simulink model "controller"  (R2024b)
settings: Solver=ode4  StartTime=0.0  StopTime=4  FixedStep=0.001  RelTol=1e-3
undefined symbols (not defined in the file): param
libraries: slpidlib x4
settings Model: Creator=mirkomizzoni  LastModifiedBy=mirkomizzoni

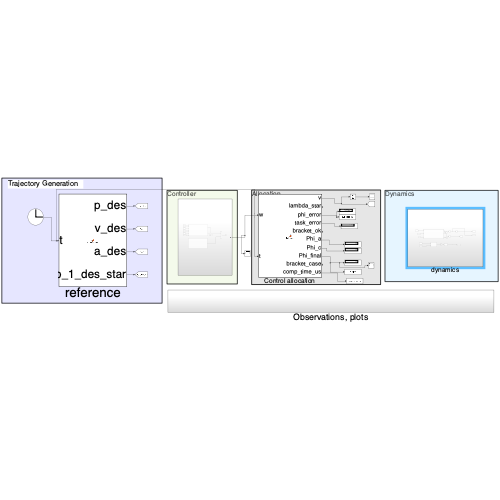
[thumbnail: Simulink's stored preview of the top-level diagram]
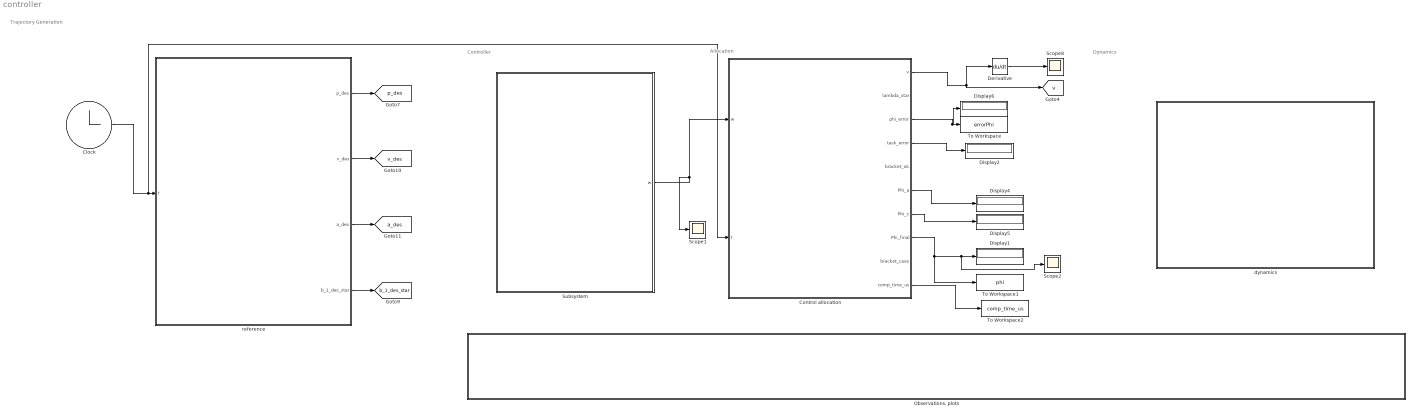
== system controller ==
  note: Trajectory Generation
  note: Dynamics
  note: Allocation
  note: Controller
  Clock : Clock
  Control allocation : MATLAB Function  TreatAsAtomicUnit=on
  Derivative : Derivative
  Display{1..2,4..6} (5 alike) : Display
  "Observations, plots" : Subsystem
  Scope1 : Scope
  Scope2 : Scope
  Scope8 : Scope
  Subsystem : Subsystem
  To Workspace : ToWorkspace  VariableName=errorPhi  SampleTime=-1
  To Workspace1 : ToWorkspace  VariableName=phi  SampleTime=-1
  To Workspace2 : ToWorkspace  VariableName=comp_time_us  SampleTime=-1
      settings: Save2DSignal=2-D array (concatenate along first dimension)
  dynamics : Subsystem
  reference : MATLAB Function  TreatAsAtomicUnit=on
  tag scope: a_des=global, b_1_des_star=global, p_des=global, v=global, v_des=global
  wires:
  reference/1(p_des) -> [p_des]
  Clock/1 -> Control allocation/2(t), reference/1(t)
  reference/3(a_des) -> [a_des]
  reference/4(b_1_des_star) -> [b_1_des_star]
  reference/2(v_des) -> [v_des]
  Control allocation/1(v) -> Derivative/1, [v]
  Derivative/1 -> Scope8/1
  Subsystem/1(w) -> Scope1/1, Control allocation/1(w)
  Control allocation/3(phi_error) -> Display6/1, To Workspace/1
  Control allocation/6(Phi_a) -> Display4/1
  Control allocation/7(Phi_c) -> Display5/1
  Control allocation/4(task_error) -> Display2/1
  Control allocation/8(Phi_final) -> To Workspace1/1, Scope2/1, Display1/1
  Control allocation/10(comp_time_us) -> To Workspace2/1

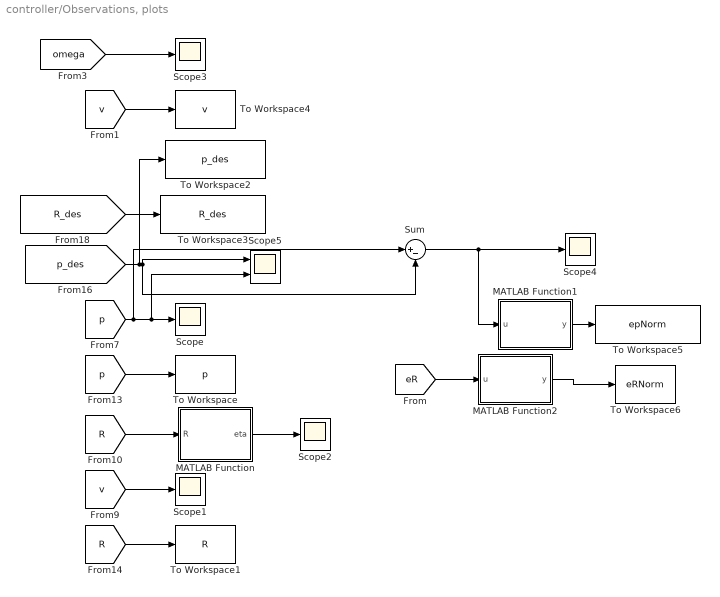
== system controller/Observations, plots ==
  MATLAB Function : MATLAB Function  TreatAsAtomicUnit=on
  MATLAB Function1 : MATLAB Function  TreatAsAtomicUnit=on
  MATLAB Function2 : MATLAB Function  TreatAsAtomicUnit=on
  Scope{,1..4} (5 alike) : Scope
  Scope5 : Scope  NumInputPorts=2
  Sum : Sum  Inputs=|+-
  To Workspace : ToWorkspace  VariableName=p  SampleTime=-1
  To Workspace1 : ToWorkspace  VariableName=R  SaveFormat=Timeseries  SampleTime=-1
  To Workspace2 : ToWorkspace  VariableName=p_des  SampleTime=-1
  To Workspace3 : ToWorkspace  VariableName=R_des  SaveFormat=Timeseries  SampleTime=-1
  To Workspace4 : ToWorkspace  VariableName=v  SampleTime=-1
  To Workspace5 : ToWorkspace  VariableName=epNorm  SampleTime=-1
  To Workspace6 : ToWorkspace  VariableName=eRNorm  SaveFormat=Timeseries  SampleTime=-1
  wires:
  [v] -> Scope1/1
  [R] -> MATLAB Function/1(R)
  [p] -> To Workspace/1
  MATLAB Function/1(eta) -> Scope2/1
  [p] -> Sum/1, Scope/1, Scope5/2
  [R] -> To Workspace1/1
  [p_des] -> Scope5/1, Sum/2, To Workspace2/1
  [R_des] -> To Workspace3/1
  [v] -> To Workspace4/1
  [omega] -> Scope3/1
  Sum/1 -> MATLAB Function1/1(u), Scope4/1
  MATLAB Function1/1(y) -> To Workspace5/1
  MATLAB Function2/1(y) -> To Workspace6/1
  [eR] -> MATLAB Function2/1(u)

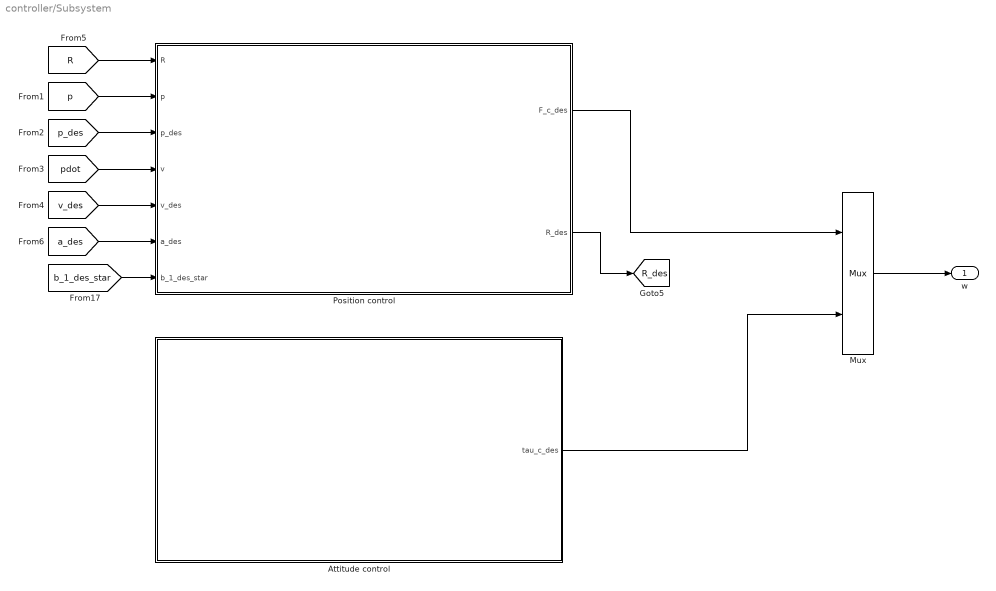
== system controller/Subsystem ==
  Attitude control : Subsystem
  Mux : Mux  Inputs=2
  Position control : Subsystem
  w : Outport
  tag scope: R_des=global
  wires:
  Position control/1(F_c_des) -> Mux/1
  Attitude control/1(tau_c_des) -> Mux/2
  [p_des] -> Position control/3(p_des)
  Position control/2(R_des) -> [R_des]
  [b_1_des_star] -> Position control/7(b_1_des_star)
  [p] -> Position control/2(p)
  [pdot] -> Position control/4(v)
  [R] -> Position control/1(R)
  Mux/1 -> w/1
  [v_des] -> Position control/5(v_des)
  [a_des] -> Position control/6(a_des)

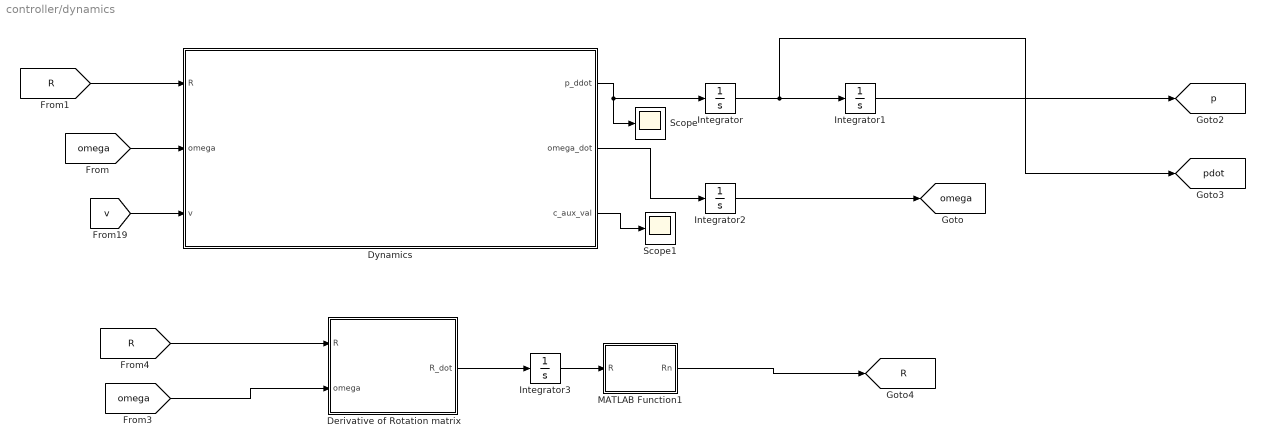
== system controller/dynamics ==
  Derivative of Rotation matrix : MATLAB Function  TreatAsAtomicUnit=on
  Dynamics : MATLAB Function  TreatAsAtomicUnit=on
  Integrator : Integrator  InitialCondition=zeros(3, 1)
  Integrator1 : Integrator  InitialCondition=[0;0.5;0]
  Integrator2 : Integrator  InitialCondition=zeros(3, 1)
  Integrator3 : Integrator  InitialCondition=param.R0
  MATLAB Function1 : MATLAB Function  TreatAsAtomicUnit=on
  Scope : Scope
  Scope1 : Scope
  tag scope: R=global, omega=global, p=global, pdot=global
  wires:
  Derivative of Rotation matrix/1(R_dot) -> Integrator3/1
  [omega] -> Dynamics/2(omega)
  Integrator2/1 -> [omega]
  Dynamics/1(p_ddot) -> Scope/1, Integrator/1
  Integrator1/1 -> [p]
  Integrator/1 -> [pdot], Integrator1/1
  Dynamics/2(omega_dot) -> Integrator2/1
  [R] -> Derivative of Rotation matrix/1(R)
  [R] -> Dynamics/1(R)
  Dynamics/3(c_aux_val) -> Scope1/1
  [v] -> Dynamics/3(v)
  Integrator3/1 -> MATLAB Function1/1(R)
  [omega] -> Derivative of Rotation matrix/2(omega)
  MATLAB Function1/1(Rn) -> [R]

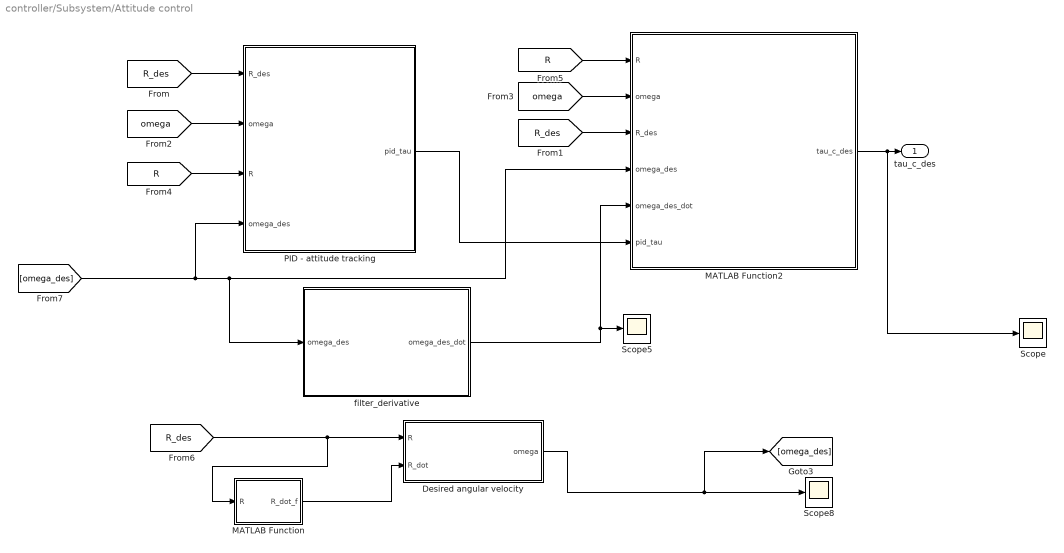
== system controller/Subsystem/Attitude control ==
  Desired angular velocity : MATLAB Function  TreatAsAtomicUnit=on
  MATLAB Function : MATLAB Function  TreatAsAtomicUnit=on
  MATLAB Function2 : MATLAB Function  TreatAsAtomicUnit=on
  PID - attitude tracking : Subsystem
  Scope : Scope
  Scope5 : Scope
  Scope8 : Scope
  filter_derivative : MATLAB Function  TreatAsAtomicUnit=on
  tau_c_des : Outport
  wires:
  MATLAB Function/1(R_dot_f) -> Desired angular velocity/2(R_dot)
  PID - attitude tracking/1(pid_tau) -> MATLAB Function2/6(pid_tau)
  MATLAB Function2/1(tau_c_des) -> Scope/1, tau_c_des/1
  filter_derivative/1(omega_des_dot) -> MATLAB Function2/5(omega_des_dot), Scope5/1
  [R_des] -> PID - attitude tracking/1(R_des)
  [R_des] -> MATLAB Function2/3(R_des)
  [omega] -> PID - attitude tracking/2(omega)
  [omega] -> MATLAB Function2/2(omega)
  [R] -> PID - attitude tracking/3(R)
  [R] -> MATLAB Function2/1(R)
  [R_des] -> MATLAB Function/1(R), Desired angular velocity/1(R)
  Desired angular velocity/1(omega) -> Scope8/1, [omega_des]
  [omega_des] -> PID - attitude tracking/4(omega_des), filter_derivative/1(omega_des), MATLAB Function2/4(omega_des)

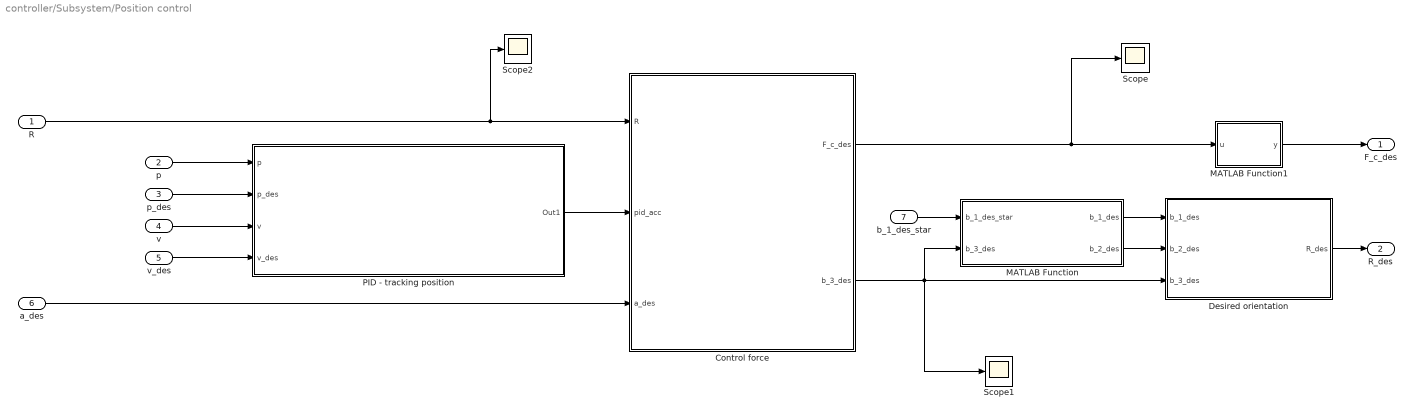
== system controller/Subsystem/Position control ==
  R : Inport
  p : Inport  Port=2
  p_des : Inport  Port=3
  v : Inport  Port=4
  v_des : Inport  Port=5
  a_des : Inport  Port=6
  b_1_des_star : Inport  Port=7
  Control force : MATLAB Function  TreatAsAtomicUnit=on
  Desired orientation : MATLAB Function  TreatAsAtomicUnit=on
  MATLAB Function : MATLAB Function  TreatAsAtomicUnit=on
  MATLAB Function1 : MATLAB Function  TreatAsAtomicUnit=on
  PID - tracking position : Subsystem
  Scope : Scope
  Scope1 : Scope
  Scope2 : Scope
  F_c_des : Outport
  R_des : Outport  Port=2
  wires:
  Control force/1(F_c_des) -> Scope/1, MATLAB Function1/1(u)
  Control force/2(b_3_des) -> Scope1/1, Desired orientation/3(b_3_des), MATLAB Function/2(b_3_des)
  R/1 -> Scope2/1, Control force/1(R)
  p_des/1 -> PID - tracking position/2(p_des)
  Desired orientation/1(R_des) -> R_des/1
  p/1 -> PID - tracking position/1(p)
  v_des/1 -> PID - tracking position/4(v_des)
  a_des/1 -> Control force/3(a_des)
  v/1 -> PID - tracking position/3(v)
  PID - tracking position/1(Out1) -> Control force/2(pid_acc)
  MATLAB Function/1(b_1_des) -> Desired orientation/1(b_1_des)
  MATLAB Function/2(b_2_des) -> Desired orientation/2(b_2_des)
  b_1_des_star/1 -> MATLAB Function/1(b_1_des_star)
  MATLAB Function1/1(y) -> F_c_des/1

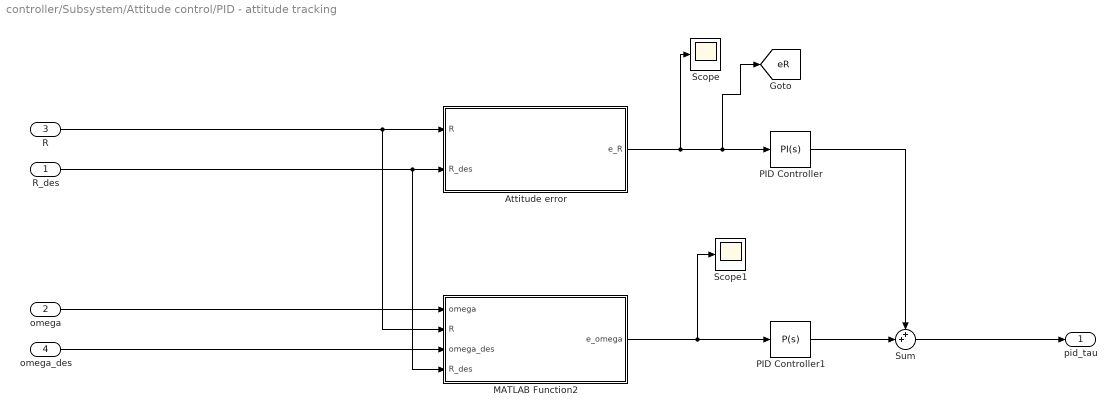
== system controller/Subsystem/Attitude control/PID - attitude tracking ==
  R_des : Inport
  omega : Inport  Port=2
  R : Inport  Port=3
  omega_des : Inport  Port=4
  Attitude error : MATLAB Function  TreatAsAtomicUnit=on
  MATLAB Function2 : MATLAB Function  TreatAsAtomicUnit=on
  PID Controller : slpidlib/PID Controller  Controller=PI  Form=Parallel  TimeDomain=Continuous-time  UseExternalTs=off  SampleTime=-1  IntegratorMethod=Forward Euler  FilterMethod=Forward Euler  ControllerParametersSource=internal  P=4*diag(param.K_tau_p)  I=[0;0;0]  UseKiTs=off  D=0  UseExternalDerivativeSource=off  N=100  UseFilter=on  TunerSelectOption=Transfer Function Based (PID Tuner App)  InitialConditionSource=internal  InitialConditionForIntegrator=0  InitialConditionForFilter=0  DifferentiatorICPrevScaledInput=0  ExternalReset=none  TrackingMode=off  Kt=1  LimitOutput=off  SatLimitsSource=internal  UpperSaturationLimit=inf  LowerSaturationLimit=-inf  LinearizeAsGain=on  AntiWindupMode=none  Kb=1  LimitIntegrator=off  UpperIntegratorSaturationLimit=inf  LowerIntegratorSaturationLimit=-inf  POutMin=[]  POutMax=[]  IOutMin=[]  IOutMax=[]  DOutMin=[]  DOutMax=[]  NOutMin=[]  NOutMax=[]  SumOutMin=[]  SumOutMax=[]  SaturationOutMin=[]  SaturationOutMax=[]  PParamMin=[]  PParamMax=[]  IParamMin=[]  IParamMax=[]  DParamMin=[]  DParamMax=[]  NParamMin=[]  NParamMax=[]  KbParamMin=[]  KbParamMax=[]  KtParamMin=[]  KtParamMax=[]  KbOutMin=[]  KbOutMax=[]  KtOutMin=[]  KtOutMax=[]  IntegratorOutMin=[]  IntegratorOutMax=[]  FilterOutMin=[]  FilterOutMax=[]  SumI1OutMin=[]  SumI1OutMax=[]  SumI2OutMin=[]  SumI2OutMax=[]  SumI3OutMin=[]  SumI3OutMax=[]  SumI4OutMin=[]  SumI4OutMax=[]  SumDOutMin=[]  SumDOutMax=[]  DifferentiatorOutMin=[]  DifferentiatorOutMax=[]  FilterDiffOutCoefMin=[]  FilterDiffOutCoefMax=[]  ReciprocalOutMin=[]  ReciprocalOutMax=[]  SumDenOutMin=[]  SumDenOutMax=[]  SumNumOutMin=[]  SumNumOutMax=[]  DivideOutMin=[]  DivideOutMax=[]  UdiffTsProdOutMin=[]  UdiffTsProdOutMax=[]  NTsProdOutMin=[]  NTsProdOutMax=[]  UintegralTsProdOutMin=[]  UintegralTsProdOutMax=[]  UngainTsProdOutMin=[]  UngainTsProdOutMax=[]  ClampingZeroOutDataTypeStr=Inherit: Inherit via back propagation  ClampingZeroOutMin=[]  ClampingZeroOutMax=[]  FilterDenConstantOutDataTypeStr=Inherit: Inherit via back propagation  FilterDenConstantOutMin=[]  FilterDenConstantOutMax=[]  PCopyOutDataTypeStr=Inherit: Inherit via back propagation  PCopyOutMin=[]  PCopyOutMax=[]  NCopyOutDataTypeStr=Inherit: Inherit via back propagation  NCopyOutMin=[]  NCopyOutMax=[]  IntegratorContinuousStateAttributes=''  IntegratorStateMustResolveToSignalObject=off  IntegratorRTWStateStorageClass=Auto  FilterContinuousStateAttributes=''  FilterStateMustResolveToSignalObject=off  FilterRTWStateStorageClass=Auto  ParallelPVariant=InternalParameters  IdealPVariant=Disabled  IVariant=InternalParameters  DVariant=Disabled  IntegratorVariant=Continuous  SatVariant=Disabled  AWVariant=Passthrough  PCopyVariant=Disabled  TRVariant=Disabled  FdbkBlocksVariant=Forward  IdealPFdbkVariant=Disabled  SatFdbkVariant=Disabled  DerivativeFilterVariant=Disabled  NVariant=Disabled  NCopyVariant=Disabled_SignalSpec  FilterICVariant=Disabled  IntegratorICVariant=InternalICs  ExternalResetVariant=Disabled  TRSumVariant=Passthrough  SumFdbkVariant=Disabled  SumVariant=Sum_PI  TsampFilterVariant=InternalTs  TsampNgainVariant=Passthrough  TsampIntegralVariant=Disabled_SignalSpec  ExternalSaturationOutDataTypeStr=Inherit: Same as second input  DerivativeSourceVariant=Disabled  PreIntVariant=InternalPreInt
  PID Controller1 : slpidlib/PID Controller  Controller=P  Form=Parallel  TimeDomain=Continuous-time  UseExternalTs=off  SampleTime=-1  IntegratorMethod=Forward Euler  FilterMethod=Forward Euler  ControllerParametersSource=internal  P=10*diag(param.K_tau_d)  I=1  UseKiTs=off  D=0  UseExternalDerivativeSource=off  N=100  UseFilter=on  TunerSelectOption=Transfer Function Based (PID Tuner App)  InitialConditionSource=internal  InitialConditionForIntegrator=0  InitialConditionForFilter=0  DifferentiatorICPrevScaledInput=0  ExternalReset=none  TrackingMode=off  Kt=1  LimitOutput=off  SatLimitsSource=internal  UpperSaturationLimit=inf  LowerSaturationLimit=-inf  LinearizeAsGain=on  AntiWindupMode=none  Kb=1  LimitIntegrator=off  UpperIntegratorSaturationLimit=inf  LowerIntegratorSaturationLimit=-inf  POutMin=[]  POutMax=[]  IOutMin=[]  IOutMax=[]  DOutMin=[]  DOutMax=[]  NOutMin=[]  NOutMax=[]  SumOutMin=[]  SumOutMax=[]  SaturationOutMin=[]  SaturationOutMax=[]  PParamMin=[]  PParamMax=[]  IParamMin=[]  IParamMax=[]  DParamMin=[]  DParamMax=[]  NParamMin=[]  NParamMax=[]  KbParamMin=[]  KbParamMax=[]  KtParamMin=[]  KtParamMax=[]  KbOutMin=[]  KbOutMax=[]  KtOutMin=[]  KtOutMax=[]  IntegratorOutMin=[]  IntegratorOutMax=[]  FilterOutMin=[]  FilterOutMax=[]  SumI1OutMin=[]  SumI1OutMax=[]  SumI2OutMin=[]  SumI2OutMax=[]  SumI3OutMin=[]  SumI3OutMax=[]  SumI4OutMin=[]  SumI4OutMax=[]  SumDOutMin=[]  SumDOutMax=[]  DifferentiatorOutMin=[]  DifferentiatorOutMax=[]  FilterDiffOutCoefMin=[]  FilterDiffOutCoefMax=[]  ReciprocalOutMin=[]  ReciprocalOutMax=[]  SumDenOutMin=[]  SumDenOutMax=[]  SumNumOutMin=[]  SumNumOutMax=[]  DivideOutMin=[]  DivideOutMax=[]  UdiffTsProdOutMin=[]  UdiffTsProdOutMax=[]  NTsProdOutMin=[]  NTsProdOutMax=[]  UintegralTsProdOutMin=[]  UintegralTsProdOutMax=[]  UngainTsProdOutMin=[]  UngainTsProdOutMax=[]  ClampingZeroOutDataTypeStr=Inherit: Inherit via back propagation  ClampingZeroOutMin=[]  ClampingZeroOutMax=[]  FilterDenConstantOutDataTypeStr=Inherit: Inherit via back propagation  FilterDenConstantOutMin=[]  FilterDenConstantOutMax=[]  PCopyOutDataTypeStr=Inherit: Inherit via back propagation  PCopyOutMin=[]  PCopyOutMax=[]  NCopyOutDataTypeStr=Inherit: Inherit via back propagation  NCopyOutMin=[]  NCopyOutMax=[]  IntegratorContinuousStateAttributes=''  IntegratorStateMustResolveToSignalObject=off  IntegratorRTWStateStorageClass=Auto  FilterContinuousStateAttributes=''  FilterStateMustResolveToSignalObject=off  FilterRTWStateStorageClass=Auto  ParallelPVariant=InternalParameters  IdealPVariant=Disabled  IVariant=Disabled  DVariant=Disabled  IntegratorVariant=Disabled  SatVariant=Disabled  AWVariant=Disabled  PCopyVariant=Disabled  TRVariant=Disabled  FdbkBlocksVariant=Forward  IdealPFdbkVariant=Disabled  SatFdbkVariant=Disabled  DerivativeFilterVariant=Disabled  NVariant=Disabled  NCopyVariant=Disabled_SignalSpec  FilterICVariant=Disabled  IntegratorICVariant=Disabled  ExternalResetVariant=Disabled  TRSumVariant=Passthrough  SumFdbkVariant=Disabled  SumVariant=Passthrough_P  TsampFilterVariant=InternalTs  TsampNgainVariant=Passthrough  TsampIntegralVariant=Disabled_SignalSpec  ExternalSaturationOutDataTypeStr=Inherit: Same as second input  DerivativeSourceVariant=Disabled  PreIntVariant=InternalPreInt
  Scope : Scope
  Scope1 : Scope
  Sum : Sum  Inputs=++|
  pid_tau : Outport
  tag scope: eR=global
  wires:
  omega/1 -> MATLAB Function2/1(omega)
  omega_des/1 -> MATLAB Function2/3(omega_des)
  PID Controller1/1 -> Sum/2
  Sum/1 -> pid_tau/1
  Attitude error/1(e_R) -> Scope/1, [eR], PID Controller/1
  MATLAB Function2/1(e_omega) -> Scope1/1, PID Controller1/1
  R/1 -> Attitude error/1(R), MATLAB Function2/2(R)
  PID Controller/1 -> Sum/1
  R_des/1 -> Attitude error/2(R_des), MATLAB Function2/4(R_des)

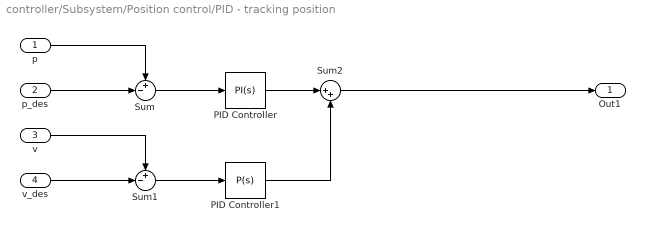
== system controller/Subsystem/Position control/PID - tracking position ==
  p : Inport
  p_des : Inport  Port=2
  v : Inport  Port=3
  v_des : Inport  Port=4
  PID Controller : slpidlib/PID Controller  Controller=PI  Form=Parallel  TimeDomain=Continuous-time  UseExternalTs=off  SampleTime=-1  IntegratorMethod=Forward Euler  FilterMethod=Forward Euler  ControllerParametersSource=internal  P=diag(param.K_F_p)  I=0*diag(param.K_F_i)  UseKiTs=off  D=0  UseExternalDerivativeSource=off  N=100  UseFilter=on  TunerSelectOption=Transfer Function Based (PID Tuner App)  InitialConditionSource=internal  InitialConditionForIntegrator=0  InitialConditionForFilter=0  DifferentiatorICPrevScaledInput=0  ExternalReset=none  TrackingMode=off  Kt=1  LimitOutput=off  SatLimitsSource=internal  UpperSaturationLimit=inf  LowerSaturationLimit=-inf  LinearizeAsGain=on  AntiWindupMode=none  Kb=1  LimitIntegrator=off  UpperIntegratorSaturationLimit=inf  LowerIntegratorSaturationLimit=-inf  POutMin=[]  POutMax=[]  IOutMin=[]  IOutMax=[]  DOutMin=[]  DOutMax=[]  NOutMin=[]  NOutMax=[]  SumOutMin=[]  SumOutMax=[]  SaturationOutMin=[]  SaturationOutMax=[]  PParamMin=[]  PParamMax=[]  IParamMin=[]  IParamMax=[]  DParamMin=[]  DParamMax=[]  NParamMin=[]  NParamMax=[]  KbParamMin=[]  KbParamMax=[]  KtParamMin=[]  KtParamMax=[]  KbOutMin=[]  KbOutMax=[]  KtOutMin=[]  KtOutMax=[]  IntegratorOutMin=[]  IntegratorOutMax=[]  FilterOutMin=[]  FilterOutMax=[]  SumI1OutMin=[]  SumI1OutMax=[]  SumI2OutMin=[]  SumI2OutMax=[]  SumI3OutMin=[]  SumI3OutMax=[]  SumI4OutMin=[]  SumI4OutMax=[]  SumDOutMin=[]  SumDOutMax=[]  DifferentiatorOutMin=[]  DifferentiatorOutMax=[]  FilterDiffOutCoefMin=[]  FilterDiffOutCoefMax=[]  ReciprocalOutMin=[]  ReciprocalOutMax=[]  SumDenOutMin=[]  SumDenOutMax=[]  SumNumOutMin=[]  SumNumOutMax=[]  DivideOutMin=[]  DivideOutMax=[]  UdiffTsProdOutMin=[]  UdiffTsProdOutMax=[]  NTsProdOutMin=[]  NTsProdOutMax=[]  UintegralTsProdOutMin=[]  UintegralTsProdOutMax=[]  UngainTsProdOutMin=[]  UngainTsProdOutMax=[]  ClampingZeroOutDataTypeStr=Inherit: Inherit via back propagation  ClampingZeroOutMin=[]  ClampingZeroOutMax=[]  FilterDenConstantOutDataTypeStr=Inherit: Inherit via back propagation  FilterDenConstantOutMin=[]  FilterDenConstantOutMax=[]  PCopyOutDataTypeStr=Inherit: Inherit via back propagation  PCopyOutMin=[]  PCopyOutMax=[]  NCopyOutDataTypeStr=Inherit: Inherit via back propagation  NCopyOutMin=[]  NCopyOutMax=[]  IntegratorContinuousStateAttributes=''  IntegratorStateMustResolveToSignalObject=off  IntegratorRTWStateStorageClass=Auto  FilterContinuousStateAttributes=''  FilterStateMustResolveToSignalObject=off  FilterRTWStateStorageClass=Auto  ParallelPVariant=InternalParameters  IdealPVariant=Disabled  IVariant=InternalParameters  DVariant=Disabled  IntegratorVariant=Continuous  SatVariant=Disabled  AWVariant=Passthrough  PCopyVariant=Disabled  TRVariant=Disabled  FdbkBlocksVariant=Forward  IdealPFdbkVariant=Disabled  SatFdbkVariant=Disabled  DerivativeFilterVariant=Disabled  NVariant=Disabled  NCopyVariant=Disabled_SignalSpec  FilterICVariant=Disabled  IntegratorICVariant=InternalICs  ExternalResetVariant=Disabled  TRSumVariant=Passthrough  SumFdbkVariant=Disabled  SumVariant=Sum_PI  TsampFilterVariant=InternalTs  TsampNgainVariant=Passthrough  TsampIntegralVariant=Disabled_SignalSpec  ExternalSaturationOutDataTypeStr=Inherit: Same as second input  DerivativeSourceVariant=Disabled  PreIntVariant=InternalPreInt
  PID Controller1 : slpidlib/PID Controller  Controller=P  Form=Parallel  TimeDomain=Continuous-time  UseExternalTs=off  SampleTime=-1  IntegratorMethod=Forward Euler  FilterMethod=Forward Euler  ControllerParametersSource=internal  P=diag(param.K_F_d)  I=1  UseKiTs=off  D=0  UseExternalDerivativeSource=off  N=100  UseFilter=on  TunerSelectOption=Transfer Function Based (PID Tuner App)  InitialConditionSource=internal  InitialConditionForIntegrator=0  InitialConditionForFilter=0  DifferentiatorICPrevScaledInput=0  ExternalReset=none  TrackingMode=off  Kt=1  LimitOutput=off  SatLimitsSource=internal  UpperSaturationLimit=inf  LowerSaturationLimit=-inf  LinearizeAsGain=on  AntiWindupMode=none  Kb=1  LimitIntegrator=off  UpperIntegratorSaturationLimit=inf  LowerIntegratorSaturationLimit=-inf  POutMin=[]  POutMax=[]  IOutMin=[]  IOutMax=[]  DOutMin=[]  DOutMax=[]  NOutMin=[]  NOutMax=[]  SumOutMin=[]  SumOutMax=[]  SaturationOutMin=[]  SaturationOutMax=[]  PParamMin=[]  PParamMax=[]  IParamMin=[]  IParamMax=[]  DParamMin=[]  DParamMax=[]  NParamMin=[]  NParamMax=[]  KbParamMin=[]  KbParamMax=[]  KtParamMin=[]  KtParamMax=[]  KbOutMin=[]  KbOutMax=[]  KtOutMin=[]  KtOutMax=[]  IntegratorOutMin=[]  IntegratorOutMax=[]  FilterOutMin=[]  FilterOutMax=[]  SumI1OutMin=[]  SumI1OutMax=[]  SumI2OutMin=[]  SumI2OutMax=[]  SumI3OutMin=[]  SumI3OutMax=[]  SumI4OutMin=[]  SumI4OutMax=[]  SumDOutMin=[]  SumDOutMax=[]  DifferentiatorOutMin=[]  DifferentiatorOutMax=[]  FilterDiffOutCoefMin=[]  FilterDiffOutCoefMax=[]  ReciprocalOutMin=[]  ReciprocalOutMax=[]  SumDenOutMin=[]  SumDenOutMax=[]  SumNumOutMin=[]  SumNumOutMax=[]  DivideOutMin=[]  DivideOutMax=[]  UdiffTsProdOutMin=[]  UdiffTsProdOutMax=[]  NTsProdOutMin=[]  NTsProdOutMax=[]  UintegralTsProdOutMin=[]  UintegralTsProdOutMax=[]  UngainTsProdOutMin=[]  UngainTsProdOutMax=[]  ClampingZeroOutDataTypeStr=Inherit: Inherit via back propagation  ClampingZeroOutMin=[]  ClampingZeroOutMax=[]  FilterDenConstantOutDataTypeStr=Inherit: Inherit via back propagation  FilterDenConstantOutMin=[]  FilterDenConstantOutMax=[]  PCopyOutDataTypeStr=Inherit: Inherit via back propagation  PCopyOutMin=[]  PCopyOutMax=[]  NCopyOutDataTypeStr=Inherit: Inherit via back propagation  NCopyOutMin=[]  NCopyOutMax=[]  IntegratorContinuousStateAttributes=''  IntegratorStateMustResolveToSignalObject=off  IntegratorRTWStateStorageClass=Auto  FilterContinuousStateAttributes=''  FilterStateMustResolveToSignalObject=off  FilterRTWStateStorageClass=Auto  ParallelPVariant=InternalParameters  IdealPVariant=Disabled  IVariant=Disabled  DVariant=Disabled  IntegratorVariant=Disabled  SatVariant=Disabled  AWVariant=Disabled  PCopyVariant=Disabled  TRVariant=Disabled  FdbkBlocksVariant=Forward  IdealPFdbkVariant=Disabled  SatFdbkVariant=Disabled  DerivativeFilterVariant=Disabled  NVariant=Disabled  NCopyVariant=Disabled_SignalSpec  FilterICVariant=Disabled  IntegratorICVariant=Disabled  ExternalResetVariant=Disabled  TRSumVariant=Passthrough  SumFdbkVariant=Disabled  SumVariant=Passthrough_P  TsampFilterVariant=InternalTs  TsampNgainVariant=Passthrough  TsampIntegralVariant=Disabled_SignalSpec  ExternalSaturationOutDataTypeStr=Inherit: Same as second input  DerivativeSourceVariant=Disabled  PreIntVariant=InternalPreInt
  Sum : Sum  Inputs=+-|
  Sum1 : Sum  Inputs=+-|
  Sum2 : Sum  Inputs=|++
  Out1 : Outport
  wires:
  v_des/1 -> Sum1/2
  v/1 -> Sum1/1
  p/1 -> Sum/1
  PID Controller/1 -> Sum2/1
  Sum2/1 -> Out1/1
  PID Controller1/1 -> Sum2/2
  Sum/1 -> PID Controller/1
  p_des/1 -> Sum/2
  Sum1/1 -> PID Controller1/1

== matlab function controller/Subsystem/Attitude control/Desired angular velocity ==
  data: R input; omega output; R_dot input
function omega = left_trans(R, R_dot)
    omega = unskew(R'*R_dot);
end

== matlab function controller/Subsystem/Attitude control/MATLAB Function2 ==
  data: R input; tau_c_des output; omega input; R_des input; omega_des input; omega_des_dot input; pid_tau input; param parameter
function tau_c_des = control_torque(R, omega, R_des, omega_des, omega_des_dot, pid_tau, param)
    J = param.J;
    tau_c_des = cross(omega, J*omega) + J*(- pid_tau + R'*R_des*omega_des_dot - cross(omega, R'*R_des*omega_des));
end

== matlab function controller/Subsystem/Attitude control/PID - attitude tracking/Attitude error ==
  data: R input; e_R output; R_des input
function e_R = error_R(R, R_des)
    e_R = 1/2*unskew(R_des'*R - R'*R_des);
end

== matlab function controller/Subsystem/Attitude control/PID - attitude tracking/MATLAB Function2 ==
  data: omega input; e_omega output; R input; omega_des input; R_des input
function e_omega = error_omega(omega, R, omega_des, R_des)
    e_omega = omega - R'*R_des*omega_des;
end

== matlab function controller/reference ==
  data: t input; p_des output; v_des output; a_des output; b_1_des_star output
function [p_des, v_des, a_des, b_1_des_star] = referenceTraj(t)
    w = pi/4;
    a = 2;
    p_des = [0.4*sin(w*t);+a*sin(w*t);0.1*sin(w*t)];
    v_des = [0.4*w*cos(w*t); a*w*cos(w*t);0.1*w*cos(w*t)];
    a_des = [-0.4*w*w*sin(w*t); a*w*w*cos(w*t);-0.1*w*w*sin(w*t)];
    b_1_des_star = [1 0 0]';
end

== matlab function controller/Subsystem/Position control/MATLAB Function ==
  data: b_1_des_star input; b_3_des input; b_1_des output; b_2_des output
function [b_1_des, b_2_des] = b_des(b_1_des_star, b_3_des)
    
    b_2_des = cross(b_3_des, b_1_des_star)/norm(cross(b_3_des, b_1_des_star));
    b_1_des = cross(b_2_des, b_3_des);
end

== matlab function controller/dynamics/MATLAB Function1 ==
  data: R input; Rn output
function Rn = fcn(R)
   [U, ~, V] = svd(R);
    Rn = U * V'; 
end

== matlab function controller/Subsystem/Attitude control/filter_derivative ==
  settings: updateMethod=DISCRETE
  data: omega_des input; omega_des_dot output
function omega_des_dot = filtered_derivative_vec3(omega_des)
% omega_des     : 3x1 desired angular velocity
% dt            : sample time
% wc            : cutoff frequency in rad/s
% omega_des_dot : filtered derivative

persistent omega_prev deriv_prev
dt = 0.001;
wc = 100;
if isempty(omega_prev)
    omega_prev = omega_des;
    deriv_prev = zeros(3,1);
end

deriv_raw = (omega_des - omega_prev) / dt;

tau = 1 / wc;
alpha = dt / (tau + dt);

omega_des_dot = deriv_prev + alpha * (deriv_raw - deriv_prev);

omega_prev = omega_des;
deriv_prev = omega_des_dot;

end

== matlab function controller/Subsystem/Attitude control/MATLAB Function ==
  settings: updateMethod=DISCRETE
  data: R input; R_dot_f output
function R_dot_f = filtered_derivative_R(R)
% R      : 3x3 rotation matrix
% dt     : sample time
% wc     : cutoff frequency in rad/s
% R_dot_f: filtered derivative of R

persistent R_prev R_dot_prev

if isempty(R_prev)
    R_prev = R;
    R_dot_prev = zeros(3,3);
end

dt = 0.001;
wc = 100;
R_dot_raw = (R - R_prev) / dt;

tau = 1 / wc;
alpha = dt / (tau + dt);

R_dot_f = R_dot_prev + alpha * (R_dot_raw - R_dot_prev);

R_prev = R;
R_dot_prev = R_dot_f;

end

== matlab function controller/Observations, plots/MATLAB Function1 ==
  data: u input; y output
function y = fcn(u)

y = norm(u);

== matlab function controller/Observations, plots/MATLAB Function2 ==
  data: u input; y output
function y = fcn(u)

y = norm(u);

== matlab function controller/Observations, plots/MATLAB Function ==
  data: R input; eta output
function eta= fcn(R)

roll = atan2(R(3,2),R(3,3));
pitch = atan2(-R(3,1),sqrt(R(3,2)^2+R(3,3)^2));
yaw = atan2(R(2,1),R(1,1));

eta = [roll;pitch;yaw];

end

== matlab function controller/dynamics/Derivative of Rotation matrix ==
  data: R input; R_dot output; omega input
function R_dot = R_dot(R, omega)
    R_dot = R*skew(omega);
end

== matlab function controller/dynamics/Dynamics ==
  data: R input; omega input; v input; p_ddot output; omega_dot output; param parameter; c_aux_val output
function [p_ddot, omega_dot, c_aux_val] = dyn(R, omega, v, param)

    e_3 = param.e_3;
    g   = param.g;
    m   = param.m;
    J   = param.J;
    Aaug = param.Aaug;

    x = v.* abs(v);
    
    w_aug_realized = Aaug*x;
   
    Fz    = w_aug_realized(1);
    tau_c = w_aug_realized(2:4);
    c_aux_val = w_aug_realized(5);

    
    F_c = [0; 0; Fz];

    p_ddot = -g*e_3 + (1/m)*R*F_c;

    omega_dot = J \ (tau_c - cross(omega, J*omega));

end

== matlab function controller/Control allocation ==
  data: w input size=[4,1]; t input; v output size=[6,1]; lambda_star output; param parameter; phi_error output; task_error output; bracket_ok output; Phi_a output; Phi_c output; Phi_final output; bracket_case output; comp_time_us output
function [v, lambda_star, phi_error, task_error, bracket_ok, Phi_a, Phi_c, Phi_final, bracket_case,comp_time_us] = OrthoAlloc(w,t, param)

% ============================================================
% OrthoAlloc
%
% Layer convention:
%   layer_id = 0      -> left extremal layer
%   layer_id = N      -> right extremal layer
%   layer_id = 1..N-1 -> intermediate layers
%
% ============================================================

coder.extrinsic('tic','toc');

comp_time_us = 0.0;

t0 = tic;


Aaug = param.Aaug;
bA = param.bA;
Cbar = param.Cbar;
layer_id = param.layer_id;

N = length(bA);

v = zeros(N,1);

rho_right_star = 0.0;
rho_left_star = 0.0;
y_transition_star = 0.0;

z = Aaug \ [w; 10000*sin(10*t)];

lambda_singular = zeros(N,1);
for i = 1:N
    lambda_singular(i) = -z(i) / bA(i);
end

lambda_sorted = sort(lambda_singular);

% ============================================================
% Solve
% ============================================================

if layer_id >= N

    lambda_N = lambda_sorted(N);

    [lambda_star, rho_right_star, phi_error, Phi_final, bracket_ok, bracket_case] = ...
        solve_right_extremal_y(bA, Cbar, lambda_singular, lambda_N);

    Phi_a = Phi_final;
    Phi_c = Phi_final;

elseif layer_id <= 0

    lambda_1 = lambda_sorted(1);

    [lambda_star, rho_left_star, phi_error, Phi_final, bracket_ok, bracket_case] = ...
        solve_left_extremal_y(bA, Cbar, lambda_singular, lambda_1);

    Phi_a = Phi_final;
    Phi_c = Phi_final;

else

    left = lambda_sorted(layer_id);
    right = lambda_sorted(layer_id + 1);

    [lambda_star, y_transition_star, phi_error, Phi_final, bracket_ok, bracket_case, Phi_a, Phi_c] = ...
        solve_transition_y(bA, Cbar, lambda_singular, left, right);

end

% ============================================================
% Recover x_alloc and v
% ============================================================

x_alloc = zeros(N,1);

if layer_id >= N

    lambda_N = lambda_sorted(N);

    for i = 1:N
        d = lambda_N - lambda_singular(i) + rho_right_star;
        x_alloc(i) = bA(i) * d;
    end

elseif layer_id <= 0

    lambda_1 = lambda_sorted(1);

    for i = 1:N
        d = lambda_1 - lambda_singular(i) - rho_left_star;
        x_alloc(i) = bA(i) * d;
    end

else

    left = lambda_sorted(layer_id);
    right = lambda_sorted(layer_id + 1);
    width = right - left;

    [q, r] = sigmoid_qr(y_transition_star);

    for i = 1:N

        if y_transition_star <= 0.0
            d = left - lambda_singular(i) + width * q;
        else
            d = right - lambda_singular(i) - width * r;
        end

        x_alloc(i) = bA(i) * d;

    end

end

for i = 1:N
    if x_alloc(i) > 0.0
        v(i) = sqrt(x_alloc(i));
    elseif x_alloc(i) < 0.0
        v(i) = -sqrt(-x_alloc(i));
    else
        v(i) = 0.0;
    end
end

% ============================================================
% Diagnostics
% ============================================================

if layer_id >= N

    Phi_final = phi_right_extremal_rho(bA, lambda_singular, lambda_sorted(N), rho_right_star);

elseif layer_id <= 0

    Phi_final = phi_left_extremal_rho(bA, lambda_singular, lambda_sorted(1), rho_left_star);

else

    Phi_final = phi_transition_y(bA, lambda_singular, lambda_sorted(layer_id), lambda_sorted(layer_id + 1), y_transition_star);

end

phi_error = abs(Phi_final - Cbar);

x_from_v = v .* abs(v);
task_error = norm(Aaug * x_from_v - [w; 0]);

elapsed = toc(t0);

comp_time_us = elapsed * 1e6;

end


function [lambda_star, rho_star, phi_error, Phi_final, bracket_ok, bracket_case] = solve_right_extremal_y(bA, Cbar, lambda_singular, lambda_N)

max_iter = 1000;
max_expand = 500;

tol_phi = 1e-10;
tol_y = 1e-12;

bracket_ok = 0;
bracket_case = 0;

lambda_star = lambda_N;
rho_star = 0.0;
Phi_final = 0.0;
phi_error = 0.0;

yL = -700.0;
yR = 10.0;

PhiL = phi_right_extremal_y(bA, lambda_singular, lambda_N, yL);
PhiR = phi_right_extremal_y(bA, lambda_singular, lambda_N, yR);

if PhiL > Cbar

    rho_star = exp(yL);
    lambda_star = lambda_N + rho_star;

    Phi_final = PhiL;
    phi_error = abs(Phi_final - Cbar);

    bracket_ok = 0;
    bracket_case = -1;
    return;

end

k = 0;
while PhiR < Cbar && k < max_expand

    yR = yR + 5.0;

    if yR > 700.0
        break;
    end

    PhiR = phi_right_extremal_y(bA, lambda_singular, lambda_N, yR);

    k = k + 1;

end

if PhiR < Cbar

    rho_star = exp(yR);
    lambda_star = lambda_N + rho_star;

    Phi_final = PhiR;
    phi_error = abs(Phi_final - Cbar);

    bracket_ok = 0;
    bracket_case = -3;
    return;

end

bracket_ok = 1;
bracket_case = 0;

for k = 1:max_iter

    yM = 0.5 * (yL + yR);
    PhiM = phi_right_extremal_y(bA, lambda_singular, lambda_N, yM);

    if abs(PhiM - Cbar) < tol_phi || abs(yR - yL) < tol_y

        rho_star = exp(yM);
        lambda_star = lambda_N + rho_star;

        Phi_final = PhiM;
        phi_error = abs(Phi_final - Cbar);
        return;

    end

    if PhiM < Cbar
        yL = yM;
    else
        yR = yM;
    end

end

yM = 0.5 * (yL + yR);

rho_star = exp(yM);
lambda_star = lambda_N + rho_star;

Phi_final = phi_right_extremal_y(bA, lambda_singular, lambda_N, yM);
phi_error = abs(Phi_final - Cbar);

end


function [lambda_star, rho_star, phi_error, Phi_final, bracket_ok, bracket_case] = solve_left_extremal_y(bA, Cbar, lambda_singular, lambda_1)

max_iter = 1000;
max_expand = 500;

tol_phi = 1e-10;
tol_y = 1e-12;

bracket_ok = 0;
bracket_case = 0;

lambda_star = lambda_1;
rho_star = 0.0;
Phi_final = 0.0;
phi_error = 0.0;

% Use -700 if you want maximum mathematical reach.
% If dynamics explode, replace by log(rho_safe), e.g. log(1e-8).
yL = -700.0;
yR = 10.0;



PhiL = phi_left_extremal_y(bA, lambda_singular, lambda_1, yL);
PhiR = phi_left_extremal_y(bA, lambda_singular, lambda_1, yR);

% Layer 0:
% PhiL near right boundary should be high.
% PhiR far left should be low.
% Need PhiR <= Cbar <= PhiL.

if PhiL < Cbar

    rho_star = exp(yL);
    lambda_star = lambda_1 - rho_star;

    Phi_final = PhiL;
    phi_error = abs(Phi_final - Cbar);

    bracket_ok = 0;
    bracket_case = -2;
    return;

end

k = 0;
while PhiR > Cbar && k < max_expand

    yR = yR + 5.0;

    if yR > 700.0
        break;
    end

    PhiR = phi_left_extremal_y(bA, lambda_singular, lambda_1, yR);

    k = k + 1;

end

if PhiR > Cbar

    rho_star = exp(yR);
    lambda_star = lambda_1 - rho_star;

    Phi_final = PhiR;
    phi_error = abs(Phi_final - Cbar);

    bracket_ok = 0;
    bracket_case = -3;
    return;

end

bracket_ok = 1;
bracket_case = 0;

for k = 1:max_iter

    yM = 0.5 * (yL + yR);
    PhiM = phi_left_extremal_y(bA, lambda_singular, lambda_1, yM);

    if abs(PhiM - Cbar) < tol_phi || abs(yR - yL) < tol_y

        rho_star = exp(yM);
        lambda_star = lambda_1 - rho_star;

        Phi_final = PhiM;
        phi_error = abs(Phi_final - Cbar);
        return;

    end

    if PhiM > Cbar
        yL = yM;
    else
        yR = yM;
    end

end

yM = 0.5 * (yL + yR);

rho_star = exp(yM);
lambda_star = lambda_1 - rho_star;

Phi_final = phi_left_extremal_y(bA, lambda_singular, lambda_1, yM);
phi_error = abs(Phi_final - Cbar);

end


function [lambda_star, y_star, phi_error, Phi_final, bracket_ok, bracket_case, Phi_a, Phi_c] = solve_transition_y(bA, Cbar, lambda_singular, left, right)

max_iter = 1000;
tol_phi = 1e-10;
tol_y = 1e-12;

lambda_star = 0.5 * (left + right);
y_star = 0.0;
phi_error = 0.0;
Phi_final = 0.0;
bracket_ok = 0;
bracket_case = 0;
Phi_a = 0.0;
Phi_c = 0.0;

width = right - left;

if width <= 0.0
    bracket_case = -9;
    return;
end

% Very near the two boundaries.
% If dynamics explode, use -30 and +30 instead.
yL = -700.0;
yR = 700.0;

Phi_a = phi_transition_y(bA, lambda_singular, left, right, yL);
Phi_c = phi_transition_y(bA, lambda_singular, left, right, yR);

if Phi_a > Cbar

    y_star = yL;
    lambda_star = lambda_from_transition_y(left, right, y_star);

    Phi_final = Phi_a;
    phi_error = abs(Phi_final - Cbar);

    bracket_ok = 0;
    bracket_case = -1;
    return;

end

if Phi_c < Cbar

    y_star = yR;
    lambda_star = lambda_from_transition_y(left, right, y_star);

    Phi_final = Phi_c;
    phi_error = abs(Phi_final - Cbar);

    bracket_ok = 0;
    bracket_case = -2;
    return;

end

bracket_ok = 1;
bracket_case = 0;

for k = 1:max_iter

    yM = 0.5 * (yL + yR);
    PhiM = phi_transition_y(bA, lambda_singular, left, right, yM);

    if abs(PhiM - Cbar) < tol_phi || abs(yR - yL) < tol_y

        y_star = yM;
        lambda_star = lambda_from_transition_y(left, right, y_star);

        Phi_final = PhiM;
        phi_error = abs(Phi_final - Cbar);
        return;

    end

    if PhiM < Cbar
        yL = yM;
    else
        yR = yM;
    end

end

y_star = 0.5 * (yL + yR);
lambda_star = lambda_from_transition_y(left, right, y_star);

Phi_final = phi_transition_y(bA, lambda_singular, left, right, y_star);
phi_error = abs(Phi_final - Cbar);

end


function Phi = phi_right_extremal_y(bA, lambda_singular, lambda_N, y)

rho = exp(y);
Phi = phi_right_extremal_rho(bA, lambda_singular, lambda_N, rho);

end


function Phi = phi_left_extremal_y(bA, lambda_singular, lambda_1, y)

rho = exp(y);
Phi = phi_left_extremal_rho(bA, lambda_singular, lambda_1, rho);

end


function Phi = phi_right_extremal_rho(bA, lambda_singular, lambda_N, rho)

n = length(bA);

eps_log = realmin;
Phi = 0.0;

for i = 1:n

    d = lambda_N - lambda_singular(i) + rho;

    ax = abs(bA(i)) * abs(d);

    if ax < eps_log
        ax = eps_log;
    end

    sx = sign(bA(i)) * sign(d);

    Phi = Phi + bA(i) * sx * log(ax);

end

end


function Phi = phi_left_extremal_rho(bA, lambda_singular, lambda_1, rho)

n = length(bA);

eps_log = realmin;
Phi = 0.0;

for i = 1:n

    d = lambda_1 - lambda_singular(i) - rho;

    ax = abs(bA(i)) * abs(d);

    if ax < eps_log
        ax = eps_log;
    end

    sx = sign(bA(i)) * sign(d);

    Phi = Phi + bA(i) * sx * log(ax);

end

end


function Phi = phi_transition_y(bA, lambda_singular, left, right, y)

n = length(bA);
width = right - left;

eps_log = realmin;
Phi = 0.0;

[q, r] = sigmoid_qr(y);

for i = 1:n

    if y <= 0.0
        d = left - lambda_singular(i) + width * q;
    else
        d = right - lambda_singular(i) - width * r;
    end

    ax = abs(bA(i)) * abs(d);

    if ax < eps_log
        ax = eps_log;
    end

    sx = sign(bA(i)) * sign(d);

    Phi = Phi + bA(i) * sx * log(ax);

end

end


function [q, r] = sigmoid_qr(y)

% q = sigmoid(y)
% r = 1 - q
%
% Computed stably.

if y >= 0.0

    ey = exp(-y);
    q = 1.0 / (1.0 + ey);
    r = ey / (1.0 + ey);

else

    ey = exp(y);
    q = ey / (1.0 + ey);
    r = 1.0 / (1.0 + ey);

end

end


function lambda = lambda_from_transition_y(left, right, y)

width = right - left;
[q, ~] = sigmoid_qr(y);

lambda = left + width * q;

end

== matlab function controller/Subsystem/Position control/MATLAB Function1 ==
  data: u input; y output
function y = fcn(u)

y = u(3);

end

== matlab function controller/Subsystem/Position control/Control force ==
  data: R input; F_c_des output; pid_acc input; a_des input; param parameter; b_3_des output
function [F_c_des, b_3_des] = control_force(R, pid_acc, a_des, param)

    m = param.m;
    g = param.g;
    e_3 = param.e_3;
    b_3 = param.b_3;

    a_cmd = -pid_acc + g*e_3 + a_des;

    b_3_des = a_cmd / norm(a_cmd);

    f = m * dot(a_cmd, R*b_3);

    F_c_des = [0; 0; f];

end

== matlab function controller/Subsystem/Position control/Desired orientation ==
  data: b_1_des input; b_2_des input; b_3_des input; R_des output
function R_des = R_star(b_1_des, b_2_des,b_3_des)
    
    R_des = [b_1_des, b_2_des, b_3_des];

end
